simulink model "ASM_Traffic_V2X_Complete_Model_2"  (R2019a)
settings: Solver=ode1  StartTime=SIM.tstart.v  StopTime=Inf  FixedStep=SIM.StepSize.v  RelTol=1e-3
PostLoadFcn:
  | if any(exist('dsrtsu_mdlpostloadfcn', 'file') ~= 0), dsrtsu_mdlpostloadfcn('Execute', bdroot); end
  | try, asm_mdl_postloadfcn(bdroot, 'UpdateModel', 2200); catch, disp(lasterr); end,
undefined symbols (not defined in the file): _SensorPnts_1, _SensorPnts_13, _SensorPnts_17, _SensorPnts_21, _SensorPnts_25, _SensorPnts_29, _SensorPnts_33, _SensorPnts_37, _SensorPnts_41, _SensorPnts_45, _SensorPnts_49, _SensorPnts_5, _SensorPnts_53, _SensorPnts_57, _SensorPnts_9, _to_, CPT, G5A, ITS, MDL, rad, s_to_rpm, SIM
libraries: simulink x169, ASM_VehicleDynamics_lib x126, ASM_Traffic_lib x83, ASM_Utils_lib x49, mdbs x45, ASM_Environment_lib x17, dspindex x12, dsaV2xLibraryAux x10, dsmpblib x6, dsaV2xAsn1Library x4, dsaV2xLibrary x4, ASM_BrakeHydraulics_lib x4
(part 11 of 36)

== system ASM_Traffic_V2X_Complete_Model_2/MDL/Drivetrain/Transmission/AutomaticTransmission ==
  Ctrl_Lockup_Clutch[%] : Inport
  Gear[] : Inport  Port=2
  n_Engine[rad|s] : Inport  Port=3
  Trq_Engine[Nm] : Inport  Port=4
  omega_In_Diff[rad|s] : Inport  Port=5
  FROM_STABILIZATION_CLUTCH : Inport  Port=6
  Reset[0|1] : Inport  Port=7
  Enable : EnablePort  PropagateVarSize=During execution
  ASMSignalCollector : Subsystem
  GEARBOX_AT : ASM_VehicleDynamics_lib/Drivetrain/Gearbox/GEARBOX_AT  Tag=ASM_SUBCOMPONENT  Map_GearRatio=MDL.Drivetrain.AutomaticTransmission.Gearbox.Map_GearRatio  Const_SyncTime=MDL.Drivetrain.AutomaticTransmission.Gearbox.Const_SyncTime  Const_Inertia_InputGear=MDL.Drivetrain.AutomaticTransmission.Gearbox.Const_Inertia_InputGear  Const_Damping_InputGear=MDL.Drivetrain.AutomaticTransmission.Gearbox.Const_Damping_InputGear  Map_Inertia_Out=MDL.Drivetrain.AutomaticTransmission.Gearbox.Map_Inertia_Out  Map_Forward_Efficiency=MDL.Drivetrain.AutomaticTransmission.Gearbox.Map_Forward_Efficiency  Map_Reverse_Efficiency=MDL.Drivetrain.AutomaticTransmission.Gearbox.Map_Reverse_Efficiency  StepSize=SIM.StepSize  ASMProperties=struct('Name','GEARBOX_AT','Version','9.0','Library','ASM_VehicleDynamics_lib')  ASMInstanceName=gearbox_at  ASMInstanceID=1
  LOCKUP_CLUTCH : ASM_VehicleDynamics_lib/Drivetrain/Clutch/LOCKUP_CLUTCH  Tag=ASM_SUBCOMPONENT  Const_Torque_Max=MDL.Drivetrain.AutomaticTransmission.Clutch.Const_Torque_Max  Map_Trq_Clutch_Red=MDL.Drivetrain.AutomaticTransmission.Clutch.Map_Trq_Clutch_Red  Const_Coef_DynamicClutchTrq=MDL.Drivetrain.AutomaticTransmission.Clutch.Const_Coef_DynamicClutchTrq  Const_Inertia=MDL.Drivetrain.AutomaticTransmission.Clutch.Const_Inertia  StepSize=SIM.StepSize  ASMProperties=struct('Name','LOCKUP_CLUTCH','Version','5.0','Library','ASM_VehicleDynamics_lib')  ASMInstanceName=TorqueConverter  ASMInstanceID=1
  SignalConversion : SignalConversion  OverrideOpt=off
  TORQUE_CONVERTER : ASM_VehicleDynamics_lib/Drivetrain/Clutch/TORQUE_CONVERTER  Tag=ASM_SUBCOMPONENT  Map_Eta_Slip=MDL.Drivetrain.AutomaticTransmission.TorqueConverter.Map_Eta_Slip  Map_Rel_Trq_PumpTurb=MDL.Drivetrain.AutomaticTransmission.TorqueConverter.Map_Rel_Trq_PumpTurb  ASMProperties=struct('Name','TORQUE_CONVERTER','Version','6.0','Library','ASM_VehicleDynamics_lib')  ASMInstanceName=TorqueConverter  ASMInstanceID=1
  Torque_Summation : Subsystem
  omega_Out_ClutchPlate_Init[rad|s] : Constant  Value=0
  ASMSignalBus : Outport
  Trq_In_Converter[Nm] : Outport  Port=2
  Trq_Out_Trm[Nm] : Outport  Port=3
  Inertia_Out_Trm[kgm2] : Outport  Port=4
  TO_STABILIZATION_GEARBOX : Outport  Port=5
  TO_STABILIZATION_CLUTCH : Outport  Port=6
  TO_STABILIZATION_TORQUE_CONVERTER : Outport  Port=7
  tag scope: ASMBUS_Drivetrain_AutomaticTransmission_Gearbox=global, ASMBUS_Drivetrain_AutomaticTransmission_LockUpClutch=global, ASMBUS_Drivetrain_AutomaticTransmission_TorqueConverter=global
  wires:
  Reset[0|1]/1 -> LOCKUP_CLUTCH/6, GEARBOX_AT/4
  ASMSignalCollector/1(ASMSignalBus) -> ASMSignalBus/1
  TORQUE_CONVERTER/2 -> Torque_Summation/3(Trq_Pump[Nm])
  LOCKUP_CLUTCH/2 -> Torque_Summation/1(Trq_Fric[Nm])
  omega_In_Diff[rad|s]/1 -> GEARBOX_AT/3
  Gear[]/1 -> GEARBOX_AT/2
  GEARBOX_AT/4 -> Inertia_Out_Trm[kgm2]/1
  GEARBOX_AT/3 -> Trq_Out_Trm[Nm]/1
  GEARBOX_AT/2 -> LOCKUP_CLUTCH/5, TORQUE_CONVERTER/2
  FROM_STABILIZATION_CLUTCH/1 -> LOCKUP_CLUTCH/4
  Ctrl_Lockup_Clutch[%]/1 -> LOCKUP_CLUTCH/3
  Trq_Engine[Nm]/1 -> LOCKUP_CLUTCH/2
  n_Engine[rad|s]/1 -> LOCKUP_CLUTCH/1, TORQUE_CONVERTER/1
  TORQUE_CONVERTER/1 -> [ASMBUS_Drivetrain_AutomaticTransmission_TorqueConverter]
  LOCKUP_CLUTCH/3 -> Torque_Summation/2(Trq_Out_LockupClutch[Nm])
  TORQUE_CONVERTER/3 -> Torque_Summation/4(Trq_Turbine[Nm])
  Torque_Summation/1(Trq_In_Converter[Nm]) -> Trq_In_Converter[Nm]/1
  Torque_Summation/2(Trq_In_Trm[Nm]) -> GEARBOX_AT/1
  GEARBOX_AT/1 -> [ASMBUS_Drivetrain_AutomaticTransmission_Gearbox]
  LOCKUP_CLUTCH/1 -> [ASMBUS_Drivetrain_AutomaticTransmission_LockUpClutch]
  GEARBOX_AT/5 -> SignalConversion/1
  TORQUE_CONVERTER/4 -> TO_STABILIZATION_TORQUE_CONVERTER/1
  LOCKUP_CLUTCH/4 -> TO_STABILIZATION_CLUTCH/1
  omega_Out_ClutchPlate_Init[rad|s]/1 -> LOCKUP_CLUTCH/7
  SignalConversion/1 -> TO_STABILIZATION_GEARBOX/1

== system ASM_Traffic_V2X_Complete_Model_2/MDL/Drivetrain/Transmission/ManualTransmission ==
  Pos_Clutch[%] : Inport
  Gear[] : Inport  Port=2
  n_Engine[rad|s] : Inport  Port=3
  Trq_Engine[Nm] : Inport  Port=4
  omega_In_Diff[rad|s] : Inport  Port=5
  FROM_STABILIZATION_CLUTCH : Inport  Port=6
  Reset[0|1] : Inport  Port=7
  Enable : EnablePort  PropagateVarSize=During execution
  ASMSignalCollector : Subsystem
  CLUTCH : ASM_VehicleDynamics_lib/Drivetrain/Clutch/CLUTCH  Tag=ASM_SUBCOMPONENT  Map_Stiffness=MDL.Drivetrain.ManualTransmission.Clutch.Map_Stiffness  Const_Damping=MDL.Drivetrain.ManualTransmission.Clutch.Const_Damping  Const_Torque_Max=MDL.Drivetrain.ManualTransmission.Clutch.Const_Torque_Max  Map_Trq_Clutch_Red=MDL.Drivetrain.ManualTransmission.Clutch.Map_Trq_Clutch_Red  Const_Coef_DynamicClutchTrq=MDL.Drivetrain.ManualTransmission.Clutch.Const_Coef_DynamicClutchTrq  Const_Inertia=MDL.Drivetrain.ManualTransmission.Clutch.Const_Inertia  StepSize=SIM.StepSize  ASMProperties=struct('Name','CLUTCH','Version','7.0','Library','ASM_VehicleDynamics_lib')  ASMInstanceName=clutch  ASMInstanceID=1
  GEARBOX_MT : ASM_VehicleDynamics_lib/Drivetrain/Gearbox/GEARBOX_MT  Tag=ASM_SUBCOMPONENT  Map_GearRatio=MDL.Drivetrain.ManualTransmission.Gearbox.Map_GearRatio  Const_SyncTime=MDL.Drivetrain.ManualTransmission.Gearbox.Const_SyncTime  Const_Inertia_InputGear=MDL.Drivetrain.ManualTransmission.Gearbox.Const_Inertia_InputGear  Const_Damping_InputGear=MDL.Drivetrain.ManualTransmission.Gearbox.Const_Damping_InputGear  Map_Inertia_Out=MDL.Drivetrain.ManualTransmission.Gearbox.Map_Inertia_Out  Map_Forward_Efficiency=MDL.Drivetrain.ManualTransmission.Gearbox.Map_Forward_Efficiency  Map_Reverse_Efficiency=MDL.Drivetrain.ManualTransmission.Gearbox.Map_Reverse_Efficiency  StepSize=SIM.StepSize  ASMProperties=struct('Name','GEARBOX_MT','Version','9.0','Library','ASM_VehicleDynamics_lib')  ASMInstanceName=gearbox_mt  ASMInstanceID=1
  SignalConversion : SignalConversion  OverrideOpt=off
  omega_Out_ClutchPlate_Init[rad|s] : Constant  Value=0
  ASMSignalBus : Outport
  Trq_Fric[Nm] : Outport  Port=2
  Trq_Out_Trm[Nm] : Outport  Port=3
  Inertia_Out_Trm[kgm2] : Outport  Port=4
  TO_STABILIZATION_GEARBOX : Outport  Port=5
  TO_STABILIZATION_CLUTCH : Outport  Port=6
  tag scope: ASMBUS_Drivetrain_ManualTransmission_Clutch=global, ASMBUS_Drivetrain_ManualTransmission_Gearbox=global
  wires:
  Reset[0|1]/1 -> GEARBOX_MT/4, CLUTCH/6
  ASMSignalCollector/1(ASMSignalBus) -> ASMSignalBus/1
  CLUTCH/3 -> GEARBOX_MT/1
  GEARBOX_MT/2 -> CLUTCH/5
  GEARBOX_MT/3 -> Trq_Out_Trm[Nm]/1
  GEARBOX_MT/4 -> Inertia_Out_Trm[kgm2]/1
  omega_In_Diff[rad|s]/1 -> GEARBOX_MT/3
  Gear[]/1 -> GEARBOX_MT/2
  n_Engine[rad|s]/1 -> CLUTCH/1
  Trq_Engine[Nm]/1 -> CLUTCH/2
  Pos_Clutch[%]/1 -> CLUTCH/3
  FROM_STABILIZATION_CLUTCH/1 -> CLUTCH/4
  GEARBOX_MT/1 -> [ASMBUS_Drivetrain_ManualTransmission_Gearbox]
  GEARBOX_MT/5 -> SignalConversion/1
  CLUTCH/4 -> TO_STABILIZATION_CLUTCH/1
  CLUTCH/1 -> [ASMBUS_Drivetrain_ManualTransmission_Clutch]
  CLUTCH/2 -> Trq_Fric[Nm]/1
  omega_Out_ClutchPlate_Init[rad|s]/1 -> CLUTCH/7
  SignalConversion/1 -> TO_STABILIZATION_GEARBOX/1

== system ASM_Traffic_V2X_Complete_Model_2/MDL/Environment/Driver/ASMSignalCollector ==
  Bus Creator : BusCreator  Inputs=4
  tag scope: ASMBUS_Environment_Driver=global
  wires:
  [ASMBUS_Env_Driver_SignalSelection] -> Bus Creator/1
  [ASMBUS_Env_Driver_LatController] -> Bus Creator/4
  [ASMBUS_Env_Driver_vRef] -> Bus Creator/3
  [ASMBUS_Env_Driver_LongController] -> Bus Creator/2
  Bus Creator/1 -> [ASMBUS_Environment_Driver]  "Driver"

== system ASM_Traffic_V2X_Complete_Model_2/MDL/Environment/Driver/LateralController ==
  Maneuver_Signals : Inport
  VehicleDynamics_Signals : Inport  Port=2
  Road_Signals : Inport  Port=3
  ASMSignalCollector : Subsystem
  Bus Creator : BusCreator  Inputs=2
  Bus Selector1 : BusSelector  OutputSignals=ModeSignals.LatDriver[1LatCtrl1|2LatCtrl2],ModeSignals.Steer_Mode[1Stim|2Driver|3Fix]
  Bus Selector2 : BusSelector  OutputSignals=Road_ASMVeh.Angle_Yaw_Veh_Road[deg],Road_ASMVeh.Pos_x_Ref_Veh_Road[m],Road_Preview.Pos_x_Preview_Road[m],Road_ASMVeh.Pos_y_Ref_Veh_Road[m],Road_Preview.Pos_y_Preview_Road[m],Road_ASMVeh.Curv_Veh_Road[1|m]
  Bus Selector3 : BusSelector  OutputSignals=VehicleMovement.Velocities.v_x_Vehicle[km|h],VehicleMovement.Velocities.v_y_Vehicle[km|h],VehicleMovement.Positions.Angle_Vehicle_CoorSys_E[x;y;z][deg].Angle_Yaw_Vehicle_CoorSys_E[deg],VehicleMovement.Velocities.YawRate_Vehicle[deg|s],VehicleMovement.Positions.Pos_Vehicle_CoorSys_E[x;y;z][m].Pos_x_Vehicle_CoorSys_E[m],VehicleMovement.Positions.Pos_Vehicle_CoorSys_E[x;y;z][m].Pos_y_Vehicle_CoorSys_E[m],Steering.i_Steering_Mean[],Tire.CorneringStiffness_Tire_Front[N|rad],Tire.CorneringStiffness_Tire_Rear[N|rad],VehicleMovement.Parameters.m_TotalVehicle[kg],VehicleMovement.Parameters.Pos_x_CoG_Vehicle_Total[m],VehicleMovement.Parameters.Inertia_z_Vehicle_Total[kgm2]
  Bus Selector4 : BusSelector  OutputSignals=Parameters.Width_Deadzone_LatCtrl[m],MdlControl.Reset_VehicleStates[0|1],ModeSignals.Steer_Mode[1Stim|2Driver|3Fix],RefSignals.Angle_SteeringWheel_Maneuver[deg],ModeSignals.LatCtrl_Mode[1Pos|2Yaw]
  LATERAL_CONTROL1 : ASM_Environment_lib/Environment/Driver/LATERAL_CONTROL1  Tag=ASM_SUBCOMPONENT  Const_t_Preview_LatCtrl=MDL.Environment.Driver.LateralController.LateralControl1.Const_t_Preview_LatCtrl  Const_t_PT1_LatCtrl=MDL.Environment.Driver.LateralController.LateralControl1.Const_t_PT1_LatCtrl  Const_WheelBase=MDL.Environment.Driver.LateralController.LateralControl1.Const_WheelBase  StepSize=SIM.StepSize  ASMProperties=struct('Name','LATERAL_CONTROL1','Version','13.0','Library','ASM_Environment_lib')  ASMInstanceName=lateral_control1  ASMInstanceID=1
  LATERAL_CONTROL2 : ASM_Environment_lib/Environment/Driver/LATERAL_CONTROL2  Tag=ASM_SUBCOMPONENT  Const_LatCtrl_kLat=MDL.Environment.Driver.LateralController.LateralControl2.Const_LatCtrl_kLat  Const_LatCtrl_kLat_i=MDL.Environment.Driver.LateralController.LateralControl2.Const_LatCtrl_kLat_i  Const_LatCtrl_kLat_Preview=MDL.Environment.Driver.LateralController.LateralControl2.Const_LatCtrl_kLat_Preview  Const_LatCtrl_kYaw=MDL.Environment.Driver.LateralController.LateralControl2.Const_LatCtrl_kYaw  Const_t_Preview_LatCtrl=MDL.Environment.Driver.LateralController.LateralControl2.Const_t_Preview_LatCtrl  Const_t_PT1_LatCtrl=MDL.Environment.Driver.LateralController.LateralControl2.Const_t_PT1_LatCtrl  Const_Kp_YawRate_Ctrl=MDL.Environment.Driver.LateralController.LateralControl2.Const_Kp_YawRate_Ctrl  Const_Ki_YawRate_Ctrl=MDL.Environment.Driver.LateralController.LateralControl2.Const_Ki_YawRate_Ctrl  StepSize=SIM.StepSize  ASMProperties=struct('Name','LATERAL_CONTROL2','Version','8.0','Library','ASM_Environment_lib')  ASMInstanceName=lateral_control2  ASMInstanceID=1
  LatCtrl1_Enable : Fcn  Expr=(u(1) == 1) * (u(2) == 2)
  LatCtrl2_Enable : Fcn  Expr=(u(1) == 2) * (u(2) == 2)
  Memory : Memory
  Multiport Switch : MultiPortSwitch  Inputs=2  SaturateOnIntegerOverflow=on
  Multiport Switch1 : MultiPortSwitch  Inputs=2  SaturateOnIntegerOverflow=on
  Mux2 : Mux  Inputs=2
  POSITION_ERRORS : ASM_Environment_lib/Environment/Driver/POSITION_ERRORS  Tag=ASM_SUBCOMPONENT  ASMProperties=struct('Name','POSITION_ERRORS','Version','1.0','Library','ASM_Environment_lib')  ASMInstanceName=position_errors  ASMInstanceID=1
  UnitConversion1 : ASM_Utils_lib/UnitConversion/UnitConversion  Selection=km/h_to_m/s
  UnitConversion2 : ASM_Utils_lib/UnitConversion/UnitConversion  Selection=km/h_to_m/s
  UnitConversion3 : ASM_Utils_lib/UnitConversion/UnitConversion  Selection=deg_to_rad
  Y_pos : Display
  laneNum : Display
  laneNumber : MATLAB Function  TreatAsAtomicUnit=on
  s_Preview_LatCtrl[m] : Outport
  Angle_SteeringWheel_LatCtrl[deg] : Outport  Port=2
  tag scope: ASMBUS_Env_Driver_LatCtrl1=global, ASMBUS_Env_Driver_LatCtrl2=global, ASMBUS_Env_Driver_LatCtrl_PosError=global
  wires:
  LatCtrl2_Enable/1 -> LATERAL_CONTROL2/1
  Bus Selector4/5 -> LATERAL_CONTROL2/18  "<LatCtrl_Mode[1Pos|2Yaw]>"
  Bus Selector2/6 -> LATERAL_CONTROL2/19  "<Curv_Veh_Road[1|m]>"
  Road_Signals/1 -> Bus Selector2/1
  Bus Selector2/1 -> LATERAL_CONTROL2/7  "<Angle_Yaw_Veh_Road[deg]>"
  Bus Selector4/4 -> LATERAL_CONTROL1/20, LATERAL_CONTROL2/16  "<Angle_SteeringWheel_Maneuver[deg]>"
  Bus Selector4/3 -> LATERAL_CONTROL1/19, LATERAL_CONTROL2/15  "<Steer_Mode[1Stim|2Driver|3Fix]>"
  Bus Selector4/2 -> LATERAL_CONTROL1/18, LATERAL_CONTROL2/14  "<Reset_VehicleStates[0|1]>"
  Bus Selector4/1 -> LATERAL_CONTROL1/17, LATERAL_CONTROL2/13  "<Width_Deadzone_LatCtrl[m]>"
  Bus Selector3/12 -> LATERAL_CONTROL1/16  "<Inertia_z_Vehicle_Total[kgm2]>"
  Bus Selector3/11 -> LATERAL_CONTROL1/15  "<Pos_x_CoG_Vehicle_Total[m]>"
  Bus Selector3/10 -> LATERAL_CONTROL1/14  "<m_TotalVehicle[kg]>"
  Memory/1 -> LATERAL_CONTROL1/13, LATERAL_CONTROL2/12
  Multiport Switch1/1 -> Memory/1, ASMSignalCollector/2(Angle_SteeringWheel_LatCtrl[deg]), Angle_SteeringWheel_LatCtrl[deg]/1
  UnitConversion3/1 -> LATERAL_CONTROL1/5, LATERAL_CONTROL2/17
  UnitConversion1/1 -> LATERAL_CONTROL1/2, LATERAL_CONTROL2/3
  LatCtrl1_Enable/1 -> LATERAL_CONTROL1/1
  Bus Selector3/4 -> UnitConversion3/1  "<YawRate_Vehicle[deg|s]>"
  Mux2/1 -> LatCtrl2_Enable/1, LatCtrl1_Enable/1
  Bus Selector1/2 -> Mux2/2  "<Steer_Mode[1Stim|2Driver|3Fix]>"
  Bus Selector3/9 -> LATERAL_CONTROL1/10  "<CorneringStiffness_Tire_Rear[N|rad]>"
  Bus Selector3/8 -> LATERAL_CONTROL1/9  "<CorneringStiffness_Tire_Front[N|rad]>"
  Bus Selector3/7 -> LATERAL_CONTROL1/8, LATERAL_CONTROL2/2  "<i_Steering_Mean[]>"
  POSITION_ERRORS/1 -> [ASMBUS_Env_Driver_LatCtrl_PosError]
  POSITION_ERRORS/2 -> ASMSignalCollector/3(e_Lat[m])
  LATERAL_CONTROL2/1 -> [ASMBUS_Env_Driver_LatCtrl2]
  LATERAL_CONTROL2/3 -> Multiport Switch1/3
  Bus Selector1/1 -> Mux2/1, Multiport Switch/1, Multiport Switch1/1  "<LatDriver[1LatCtrl1|2LatCtrl2]>"
  Maneuver_Signals/1 -> Bus Selector1/1, Bus Selector4/1
  UnitConversion2/1 -> LATERAL_CONTROL1/3
  Bus Selector3/5 -> LATERAL_CONTROL1/6, POSITION_ERRORS/2, LATERAL_CONTROL2/5  "<Pos_x_Vehicle_CoorSys_E[m]>"
  Bus Selector3/3 -> LATERAL_CONTROL1/4, POSITION_ERRORS/1, LATERAL_CONTROL2/4  "<Angle_Yaw_Vehicle_CoorSys_E[deg]>"
  Bus Selector3/2 -> UnitConversion2/1  "<v_y_Vehicle[km|h]>"
  Bus Selector3/1 -> UnitConversion1/1  "<v_x_Vehicle[km|h]>"
  Bus Selector2/4 -> LATERAL_CONTROL2/10, POSITION_ERRORS/5  "<Pos_y_Ref_Veh_Road[m]>"
  Bus Selector2/2 -> LATERAL_CONTROL2/8, POSITION_ERRORS/4  "<Pos_x_Ref_Veh_Road[m]>"
  VehicleDynamics_Signals/1 -> Bus Selector3/1
  LATERAL_CONTROL1/3 -> Multiport Switch1/2
  LATERAL_CONTROL1/2 -> Multiport Switch/2
  LATERAL_CONTROL2/2 -> Multiport Switch/3
  Multiport Switch/1 -> ASMSignalCollector/1(s_Preview_LatCtrl[m]), s_Preview_LatCtrl[m]/1
  Bus Selector2/5 -> LATERAL_CONTROL1/12, LATERAL_CONTROL2/11  "<Pos_y_Preview_Road[m]>"
  Bus Selector2/3 -> LATERAL_CONTROL1/11, LATERAL_CONTROL2/9  "<Pos_x_Preview_Road[m]>"
  laneNumber/1(laneNumber) -> Bus Creator/1, laneNum/1
  LATERAL_CONTROL1/1 -> Bus Creator/2
  Bus Selector3/6 -> Y_pos/1, laneNumber/1(u), LATERAL_CONTROL1/7, POSITION_ERRORS/3, LATERAL_CONTROL2/6  "<Pos_y_Vehicle_CoorSys_E[m]>"
  Bus Creator/1 -> [ASMBUS_Env_Driver_LatCtrl1]

== system ASM_Traffic_V2X_Complete_Model_2/MDL/Environment/Driver/LongitudinalController ==
  Maneuver_Signals : Inport
  Drivetrain_Signals : Inport  Port=2
  SoftECU_Engine_Signals : Inport  Port=3
  VehicleDynamics_Signals : Inport  Port=4
  v_Vehicle_Ref[m|s] : Inport  Port=5
  v_Vehicle_Ref_Preview[m|s] : Inport  Port=6
  ASMSignalCollector : Subsystem
  Bus Selector1 : BusSelector  OutputSignals=Parameters.Gear_Max[],RefSignals.Pos_AccPedal_Maneuver[%],RefSignals.Pos_BrakePedal_Maneuver[%],ModeSignals.AccBr_Mode[1Stim|2Driver],RefSignals.Gear_Maneuver[],RefSignals.Pos_ClutchPedal_Maneuver[%],ModeSignals.GearClutch_Mode[1Stim|2Driver|3OpenClutch|4RefGear],RefSignals.SelectorLever_Maneuver[],ModeSignals.SelectorLever_Mode[1Stim|2Driver],MdlControl.Reset_VehicleStates[0|1]
  Bus Selector2 : BusSelector  OutputSignals=VehicleMovement.Parameters.m_TotalVehicle[kg]
  Bus Selector3 : BusSelector  OutputSignals=n_Engine[rpm],omega_Out_Trm[rad|s]
  Bus Selector4 : BusSelector  OutputSignals=VehicleMovement.Velocities.v_x_Vehicle[km|h]
  Bus Selector5 : BusSelector  OutputSignals=SoftECU_Engine.State_Engine[0|1|2|3|4],SoftECU_Engine.Const_n_Engine_Idle_Set[rpm]
  Bus Selector6 : BusSelector  OutputSignals=ModeSignals.AccBr_Mode[1Stim|2Driver],RefSignals.Pos_AccPedal_Maneuver[%],RefSignals.Pos_BrakePedal_Maneuver[%],MdlControl.Reset_VehicleStates[0|1]
  Default_GearClutch_Mode : Subsystem
      mask Display: disp('Default GearClutch_Mode')
  Driving_Resistances : Subsystem
  GEAR_SHIFTER : ASM_Environment_lib/Environment/Driver/GEAR_SHIFTER  Tag=ASM_SUBCOMPONENT  Map_Gear_StartUp=MDL.Environment.Driver.LongitudinalController.GearShifter.Map_Gear_StartUp  Const_n_Engine_StartUp_Set=MDL.Environment.Driver.LongitudinalController.GearShifter.Const_n_Engine_StartUp_Set  Const_P_Gain_StartUp=MDL.Environment.Driver.LongitudinalController.GearShifter.Const_P_Gain_StartUp  Const_I_Gain_StartUp=MDL.Environment.Driver.LongitudinalController.GearShifter.Const_I_Gain_StartUp  Const_D_Gain_StartUp=MDL.Environment.Driver.LongitudinalController.GearShifter.Const_D_Gain_StartUp  Const_a_x_Vehicle_UpLim=MDL.Environment.Driver.LongitudinalController.GearShifter.Const_a_x_Vehicle_UpLim  Const_a_Tractive_Res_UpLim=MDL.Environment.Driver.LongitudinalController.GearShifter.Const_a_Tractive_Res_UpLim  Const_v_x_Vehicle_LowLim=MDL.Environment.Driver.LongitudinalController.GearShifter.Const_v_x_Vehicle_LowLim  Const_a_x_Vehicle_LowLim=MDL.Environment.Driver.LongitudinalController.GearShifter.Const_a_x_Vehicle_LowLim  Const_t_Gear_Neutral=MDL.Environment.Driver.LongitudinalController.GearShifter.Const_t_Gear_Neutral  Const_t_Hold_ClutchPedal=MDL.Environment.Driver.LongitudinalController.GearShifter.Const_t_Hold_ClutchPedal  Map_Pos_AccPedal=MDL.Environment.Driver.LongitudinalController.GearShifter.Map_Pos_AccPedal  Const_P_Gain_ClutchPedal=MDL.Environment.Driver.LongitudinalController.GearShifter.Const_P_Gain_ClutchPedal  Const_I_Gain_ClutchPedal=MDL.Environment.Driver.LongitudinalController.GearShifter.Const_I_Gain_ClutchPedal  Map_Pos_ClutchPedal_Disengagement_StartUp=MDL.Environment.Driver.LongitudinalController.GearShifter.Map_Pos_ClutchPedal_Disengagement_StartUp  Map_Pos_ClutchPedal_Disengagement=MDL.Environment.Driver.LongitudinalController.GearShifter.Map_Pos_ClutchPedal_Disengagement  Map_Pos_ClutchPedal_Engagement_StartUp=MDL.Environment.Driver.LongitudinalController.GearShifter.Map_Pos_ClutchPedal_Engagement_StartUp  Map_Pos_ClutchPedal_Engagement=MDL.Environment.Driver.LongitudinalController.GearShifter.Map_Pos_ClutchPedal_Engagement  Map_n_Engine_Upshift_Lim=MDL.Environment.Driver.LongitudinalController.GearShifter.Map_n_Engine_Upshift_Lim  Map_n_Engine_Downshift_Lim=MDL.Environment.Driver.LongitudinalController.GearShifter.Map_n_Engine_Downshift_Lim  Map_omega_Out_Trm_Shift_Bias=MDL.Environment.Driver.LongitudinalController.GearShifter.Map_omega_Out_Trm_Shift_Bias  Map_i_Ratio=MDL.Environment.Driver.LongitudinalController.GearShifter.Map_i_Ratio  Sw_Upshift_Gear_Skipping=MDL.Environment.Driver.LongitudinalController.GearShifter.Sw_Upshift_Gear_Skipping  Sw_ClutchPedal_EngineOff=MDL.Environment.Driver.LongitudinalController.GearShifter.Sw_ClutchPedal_EngineOff  StepSize=SIM.StepSize  ASMProperties=struct('Name','GEAR_SHIFTER','Version','17.0','Library','ASM_Environment_lib')  ASMInstanceName=gear_shifter  ASMInstanceID=1
  Gear_Min_Maneuver[0Off|-n_-1] : Constant  Value=0
  LONGITUDINAL_CONTROL : ASM_Environment_lib/Environment/Driver/LONGITUDINAL_CONTROL  Tag=ASM_SUBCOMPONENT  Map_P_vCtrl=MDL.Environment.Driver.LongitudinalController.LongControl.Map_P_vCtrl  Map_I_vCtrl=MDL.Environment.Driver.LongitudinalController.LongControl.Map_I_vCtrl  Const_P_FeedForward_aCtrl=MDL.Environment.Driver.LongitudinalController.LongControl.Const_P_FeedForward_aCtrl  Const_Pos_BrakePedal_Standstill=MDL.Environment.Driver.LongitudinalController.LongControl.Const_Pos_BrakePedal_Standstill  Const_t_Min_Pedals=MDL.Environment.Driver.LongitudinalController.LongControl.Const_t_Min_Pedals  Const_Max_AccPedal=MDL.Environment.Driver.LongitudinalController.LongControl.Const_Max_AccPedal  Const_Rate_Rise_Max_AccPedal=MDL.Environment.Driver.LongitudinalController.LongControl.Const_Rate_Rise_Max_AccPedal  Const_Rate_Drop_Max_AccPedal=MDL.Environment.Driver.LongitudinalController.LongControl.Const_Rate_Drop_Max_AccPedal  Const_Max_BrakePedal=MDL.Environment.Driver.LongitudinalController.LongControl.Const_Max_BrakePedal  Const_Rate_Rise_Max_BrakePedal=MDL.Environment.Driver.LongitudinalController.LongControl.Const_Rate_Rise_Max_BrakePedal  Const_Rate_Drop_Max_BrakePedal=MDL.Environment.Driver.LongitudinalController.LongControl.Const_Rate_Drop_Max_BrakePedal  Const_t_Preview=MDL.Environment.Driver.LongitudinalController.LongControl.Const_t_Preview  StepSize=SIM.StepSize  ASMProperties=struct('Name','LONGITUDINAL_CONTROL','Version','3.0','Library','ASM_Environment_lib')  ASMInstanceName=longitudinal_control  ASMInstanceID=1
  No_StartStop : Constant
  Running_Engine : Constant  Value=3
  UnitConversion : ASM_Utils_lib/UnitConversion/UnitConversion  Selection=km/h_to_m/s
  Pos_AccPedal[%] : Outport
  Pos_BrakePedal[%] : Outport  Port=2
  Pos_ClutchPedal[%] : Outport  Port=3
  Gear[] : Outport  Port=4
  SelectorLever[-3T|-2P|-1R|0N|1D] : Outport  Port=5
  t_Preview_vRef[s] : Outport  Port=6
  tag scope: ASMBUS_Env_Driver_GearShifter=global, ASMBUS_Env_Driver_LongCtrl=global
  wires:
  Running_Engine/1 -> LONGITUDINAL_CONTROL/8
  LONGITUDINAL_CONTROL/2 -> t_Preview_vRef[s]/1
  v_Vehicle_Ref_Preview[m|s]/1 -> GEAR_SHIFTER/24, LONGITUDINAL_CONTROL/3
  Bus Selector6/4 -> LONGITUDINAL_CONTROL/7  "<Reset_VehicleStates[0|1]>"
  Bus Selector6/3 -> LONGITUDINAL_CONTROL/6  "<Pos_BrakePedal_Maneuver[%]>"
  Bus Selector6/2 -> LONGITUDINAL_CONTROL/5  "<Pos_AccPedal_Maneuver[%]>"
  Bus Selector6/1 -> LONGITUDINAL_CONTROL/4  "<AccBr_Mode[1Stim|2Driver]>"
  Bus Selector3/2 -> GEAR_SHIFTER/9  "<omega_Out_Trm[rad|s]>"
  Driving_Resistances/1(F_Tractive_Res[N]) -> GEAR_SHIFTER/4
  No_StartStop/1 -> GEAR_SHIFTER/23, LONGITUDINAL_CONTROL/9
  Default_GearClutch_Mode/1(GearClutch_Mode[1Stim|2Driver|3OpenClutch|4RefGear]_) -> GEAR_SHIFTER/19
  GEAR_SHIFTER/6 -> SelectorLever[-3T|-2P|-1R|0N|1D]/1
  GEAR_SHIFTER/5 -> Gear[]/1
  GEAR_SHIFTER/4 -> Pos_ClutchPedal[%]/1
  GEAR_SHIFTER/3 -> Pos_BrakePedal[%]/1
  GEAR_SHIFTER/2 -> Pos_AccPedal[%]/1
  Bus Selector1/9 -> GEAR_SHIFTER/21  "<SelectorLever_Mode[1Stim|2Driver]>"
  Bus Selector1/8 -> GEAR_SHIFTER/20  "<SelectorLever_Maneuver[]>"
  Bus Selector1/7 -> Default_GearClutch_Mode/1(GearClutch_Mode[1Stim|2Driver|3OpenClutch|4RefGear])  "<GearClutch_Mode[1Stim|2Driver|3OpenClutch|4RefGear]>"
  Bus Selector1/6 -> GEAR_SHIFTER/18  "<Pos_ClutchPedal_Maneuver[%]>"
  Bus Selector1/5 -> GEAR_SHIFTER/17  "<Gear_Maneuver[]>"
  Bus Selector1/4 -> GEAR_SHIFTER/16  "<AccBr_Mode[1Stim|2Driver]>"
  Bus Selector1/3 -> GEAR_SHIFTER/15  "<Pos_BrakePedal_Maneuver[%]>"
  Bus Selector1/2 -> GEAR_SHIFTER/14  "<Pos_AccPedal_Maneuver[%]>"
  Bus Selector1/1 -> GEAR_SHIFTER/13  "<Gear_Max[]>"
  Bus Selector5/2 -> GEAR_SHIFTER/11  "<Const_n_Engine_Idle_Set[rpm]>"
  Bus Selector5/1 -> GEAR_SHIFTER/10  "<State_Engine[0|1|2|3|4]>"
  Gear_Min_Maneuver[0Off|-n_-1]/1 -> GEAR_SHIFTER/12
  LONGITUDINAL_CONTROL/3 -> GEAR_SHIFTER/2
  GEAR_SHIFTER/1 -> [ASMBUS_Env_Driver_GearShifter]
  LONGITUDINAL_CONTROL/1 -> [ASMBUS_Env_Driver_LongCtrl]
  SoftECU_Engine_Signals/1 -> Bus Selector5/1
  Bus Selector1/10 -> GEAR_SHIFTER/22  "<Reset_VehicleStates[0|1]>"
  Bus Selector2/1 -> GEAR_SHIFTER/8  "<m_TotalVehicle[kg]>"
  UnitConversion/1 -> GEAR_SHIFTER/5, LONGITUDINAL_CONTROL/1
  Maneuver_Signals/1 -> Bus Selector6/1, Bus Selector1/1
  Bus Selector3/1 -> GEAR_SHIFTER/7  "<n_Engine[rpm]>"
  Drivetrain_Signals/1 -> Bus Selector3/1
  LONGITUDINAL_CONTROL/4 -> GEAR_SHIFTER/3
  [TAG_Sw_Transmission_Mode] -> GEAR_SHIFTER/1
  Bus Selector4/1 -> UnitConversion/1  "<v_x_Vehicle[km|h]>"
  VehicleDynamics_Signals/1 -> Bus Selector4/1, Bus Selector2/1, Driving_Resistances/1(VehicleDynamics_Signals)
  v_Vehicle_Ref[m|s]/1 -> GEAR_SHIFTER/6, LONGITUDINAL_CONTROL/2

== system ASM_Traffic_V2X_Complete_Model_2/MDL/Environment/Driver/ReferenceVelocity ==
  Maneuver_Signals : Inport
  VehicleDynamics_Signals : Inport  Port=2
  Road_Signals : Inport  Port=3
  Bus Selector1 : BusSelector  OutputSignals=RefSignals.v_Vehicle_Ref_Preview_Maneuver[m|s]
  Bus Selector2 : BusSelector  OutputSignals=VehicleMovement.Velocities.v_x_Vehicle[km|h]
  Bus Selector3 : BusSelector  OutputSignals=MdlControl.Reset_VehicleStates[0|1],ModeSignals.AccBr_Mode[1Stim|2Driver]
  Bus Selector4 : BusSelector  OutputSignals=Road_ASMVeh.s_Veh_Road[m],Road_Preview.Pitch_Preview_Road[deg],Road_Preview.Pos_z_Preview_Road[m]
  Bus Selector5 : BusSelector  OutputSignals=Road_Info.Speed_Limit_Veh[km|h],Road_Preview.Speed_Limit_Preview_Road[km|h]
  Bus Selector6 : BusSelector  OutputSignals=Road_Info.Dist_Border_Left[m],Road_Info.Dist_Border_Right[m]
  Bus Selector7 : BusSelector  OutputSignals=Road_Preview.x_Preview_DriverCurv[m],Road_Preview.y_Preview_DriverCurv[m],Road_ASMVeh.Curv_Veh_Road[1|m],Road_Preview.Curv_Preview_Road[1|m]
  Bus Selector8 : BusSelector  OutputSignals=ModeSignals.AdaptVelocityToRoad_Mode[1Off|2On],RefSignals.v_Vehicle_Ref_Maneuver[m|s],Parameters.a_x_Max[m|s2],Parameters.a_x_Brake_Threshold[m|s2],Parameters.a_y_Max[m|s2]
  Bus Selector9 : BusSelector  OutputSignals=ModeSignals.CurvatureCalculation_Mode[1Road|2Driver]
  Curves_are_not_considered : Gain
  DRIVER_CURVATURE : ASM_Environment_lib/Environment/Driver/DRIVER_CURVATURE  Tag=ASM_SUBCOMPONENT  ASMProperties=struct('Name','DRIVER_CURVATURE','Version','1.0','Library','ASM_Environment_lib')  ASMInstanceName=driver_curvature  ASMInstanceID=1
  Extend_Dimension : Subsystem
  Reduce_Dimension2 : Subsystem
  Reduce_Dimension3 : Subsystem
  Reduce_Dimension4 : Subsystem
  Reduce_Dimension5 : Subsystem
  Terminator : Terminator
  Terminator_2 : Terminator
  UnitConversion : ASM_Utils_lib/UnitConversion/UnitConversion  Selection=km/h_to_m/s
  UnitConversion1 : ASM_Utils_lib/UnitConversion/UnitConversion  Selection=km/h_to_m/s
  UnitConversion4 : ASM_Utils_lib/UnitConversion/UnitConversion  Selection=km/h_to_m/s
  V_ROAD_REF : ASM_Environment_lib/Environment/Driver/V_ROAD_REF  Tag=ASM_SUBCOMPONENT  StepSize=SIM.StepSize  ASMProperties=struct('Name','V_ROAD_REF','Version','7.0','Library','ASM_Environment_lib')  ASMInstanceName=v_road_ref  ASMInstanceID=1
  a_z_Max_Deflect[m|s2] : Constant  Value=2.5
  a_z_Max_Rebound[m|s2] : Constant  Value=-3.5
  v_Vehicle_Ref[m|s] : Outport
  v_Vehicle_Ref_Preview[m|s] : Outport  Port=2
  s_Preview_vRef[m] : Outport  Port=3
  tag scope: ASMBUS_Env_Driver_GetCurvature=global, ASMBUS_Env_Driver_vRef=global
  wires:
  Reduce_Dimension5/1(Out) -> DRIVER_CURVATURE/5
  Bus Selector7/1 -> DRIVER_CURVATURE/2  "<x_Preview_DriverCurv[m]>"
  Bus Selector7/2 -> DRIVER_CURVATURE/3  "<y_Preview_DriverCurv[m]>"
  Bus Selector7/4 -> Reduce_Dimension5/1(In)  "<Curv_Preview_Road[1|m]>"
  Bus Selector7/3 -> DRIVER_CURVATURE/4  "<Curv_Veh_Road[1|m]>"
  Road_Signals/1 -> Bus Selector5/1, Bus Selector4/1, Bus Selector6/1, Bus Selector7/1
  Maneuver_Signals/1 -> Bus Selector1/1, Bus Selector9/1, Bus Selector3/1, Bus Selector8/1
  Bus Selector9/1 -> DRIVER_CURVATURE/1  "<CurvatureCalculation_Mode[1Road|2Driver]>"
  [ASMBUS_Env_Driver_GetCurvature] -> Terminator_2/1
  DRIVER_CURVATURE/3 -> V_ROAD_REF/8
  DRIVER_CURVATURE/2 -> V_ROAD_REF/7
  DRIVER_CURVATURE/1 -> [ASMBUS_Env_Driver_GetCurvature]
  Bus Selector6/2 -> V_ROAD_REF/19  "<Dist_Border_Right[m]>"
  Bus Selector6/1 -> V_ROAD_REF/18  "<Dist_Border_Left[m]>"
  V_ROAD_REF/4 -> Extend_Dimension/1(In)
  V_ROAD_REF/3 -> v_Vehicle_Ref[m|s]/1
  V_ROAD_REF/2 -> Terminator/1
  V_ROAD_REF/1 -> [ASMBUS_Env_Driver_vRef]
  Reduce_Dimension4/1(Out) -> V_ROAD_REF/15
  Reduce_Dimension3/1(Out) -> V_ROAD_REF/14
  a_z_Max_Deflect[m|s2]/1 -> V_ROAD_REF/17
  a_z_Max_Rebound[m|s2]/1 -> V_ROAD_REF/16
  Bus Selector4/3 -> Reduce_Dimension4/1(In)  "<Pos_z_Preview_Road[m]>"
  Bus Selector4/2 -> Reduce_Dimension3/1(In)  "<Pitch_Preview_Road[deg]>"
  Bus Selector4/1 -> V_ROAD_REF/13  "<s_Veh_Road[m]>"
  Bus Selector3/2 -> V_ROAD_REF/12  "<AccBr_Mode[1Stim|2Driver]>"
  Bus Selector3/1 -> V_ROAD_REF/11  "<Reset_VehicleStates[0|1]>"
  Bus Selector5/2 -> UnitConversion4/1  "<Speed_Limit_Preview_Road[km|h]>"
  Bus Selector5/1 -> UnitConversion/1  "<Speed_Limit_Veh[km|h]>"
  Bus Selector8/1 -> V_ROAD_REF/1  "<AdaptVelocityToRoad_Mode[1Off|2On]>"
  Bus Selector8/5 -> V_ROAD_REF/5  "<a_y_Max[m|s2]>"
  Bus Selector8/4 -> V_ROAD_REF/4  "<a_x_Brake_Threshold[m|s2]>"
  Bus Selector8/3 -> V_ROAD_REF/3  "<a_x_Max[m|s2]>"
  UnitConversion1/1 -> V_ROAD_REF/6
  Bus Selector2/1 -> UnitConversion1/1  "<v_x_Vehicle[km|h]>"
  Bus Selector8/2 -> V_ROAD_REF/2  "<v_Vehicle_Ref_Maneuver[m|s]>"
  UnitConversion4/1 -> Reduce_Dimension2/1(In)
  UnitConversion/1 -> V_ROAD_REF/9
  VehicleDynamics_Signals/1 -> Bus Selector2/1
  Extend_Dimension/1(Out) -> s_Preview_vRef[m]/1
  Reduce_Dimension2/1(Out) -> V_ROAD_REF/10
  Curves_are_not_considered/1 -> v_Vehicle_Ref_Preview[m|s]/1
  Bus Selector1/1 -> Curves_are_not_considered/1  "<v_Vehicle_Ref_Preview_Maneuver[m|s]>"

== system ASM_Traffic_V2X_Complete_Model_2/MDL/Environment/Driver/SignalSelection ==
  Maneuver_Signals : Inport
  Pos_AccPedal[%] : Inport  Port=2
  Pos_BrakePedal[%] : Inport  Port=3
  Pos_ClutchPedal[%] : Inport  Port=4
  Gear[] : Inport  Port=5
  SelectorLever_Driver[-3T|-2P|-1R|0N|1D] : Inport  Port=6
  t_Preview_vRef[s] : Inport  Port=7
  Angle_SteeringWheel[deg] : Inport  Port=8
  ASMSignalCollector : Subsystem
  Bus Creator : BusCreator  Inputs=2
  Bus Creator2 : BusCreator  Inputs=9
  Bus Selector3 : BusSelector  OutputSignals=TipShiftSignals.SW_TipTronic[-1Down|0Off|1Up],StartButtonSignals,ParkingBrakeSignals
  Driver_Signals : Outport
  wires:
  t_Preview_vRef[s]/1 -> Bus Creator2/5  "t_Preview_vRef[s]"
  Bus Creator2/1 -> Driver_Signals/1, ASMSignalCollector/1(Driver_Signals)  "Driver"
  Bus Selector3/3 -> Bus Creator2/9  "<ParkingBrakeSignals>"
  Bus Selector3/1 -> Bus Creator/2  "<SW_TipTronic[-1Down|0Off|1Up]>"
  SelectorLever_Driver[-3T|-2P|-1R|0N|1D]/1 -> Bus Creator/1  "SelectorLever[-3T|-2P|-1R|0N|1D]"
  Bus Creator/1 -> Bus Creator2/7  "AutomaticTrmCtrlSignals"
  Pos_BrakePedal[%]/1 -> Bus Creator2/2  "Pos_BrakePedal[%]"
  Pos_AccPedal[%]/1 -> Bus Creator2/1  "Pos_AccPedal[%]"
  Bus Selector3/2 -> Bus Creator2/8  "<StartButtonSignals>"
  Pos_ClutchPedal[%]/1 -> Bus Creator2/3  "Pos_ClutchPedal[%]"
  Angle_SteeringWheel[deg]/1 -> Bus Creator2/6  "Angle_SteeringWheel[deg]"
  Gear[]/1 -> Bus Creator2/4  "Gear[]"
  Maneuver_Signals/1 -> Bus Selector3/1

== system ASM_Traffic_V2X_Complete_Model_2/MDL/Environment/Driver/Source_of_eGoCAR_Control_Conditions ==
  note: SteeringAngle
  note: Break
  note: Throttle
  In1 : Inport
  Throttle_Input_SIM : Inport  Port=2
  Break_Input_SIM : Inport  Port=3
  Steering_Input_SIM : Inport  Port=4
  eGOCAR_Speed_kmh : Inport  Port=5
  Break_Switch_Value : Constant
  Bus Selector : BusSelector  OutputSignals=signal1,signal2,signal3
  Steer_Decision_Conditions : Subsystem
  Steer_Switch_Value : Constant
  Switch_Break : Switch  Criteria=u2 > Threshold
  Switch_Steer : Switch  Criteria=u2 > Threshold
  Switch_Throtle : Switch  Criteria=u2 > Threshold
  Terminator1 : Terminator
  Throtle_Switch_Value : Constant
  Throttle : Outport
  Break : Outport  Port=2
  Steering : Outport  Port=3
  wires:
  In1/1 -> Bus Selector/1
  Bus Selector/3 -> Switch_Steer/3  "<signal3>"
  Bus Selector/2 -> Switch_Break/3  "<signal2>"
  Bus Selector/1 -> Switch_Throtle/3  "<signal1>"
  Throttle_Input_SIM/1 -> Switch_Throtle/1
  Throtle_Switch_Value/1 -> Switch_Throtle/2
  Break_Switch_Value/1 -> Switch_Break/2
  Steer_Switch_Value/1 -> Switch_Steer/2
  Steering_Input_SIM/1 -> Switch_Steer/1
  Break_Input_SIM/1 -> Switch_Break/1
  Switch_Throtle/1 -> Throttle/1
  Switch_Break/1 -> Break/1
  Switch_Steer/1 -> Steering/1
  eGOCAR_Speed_kmh/1 -> Steer_Decision_Conditions/1(In1)
  Steer_Decision_Conditions/1(Out1) -> Terminator1/1

== system ASM_Traffic_V2X_Complete_Model_2/MDL/Environment/Driver/SteeringWheelAngle_Control ==
  SteerWheelAngle_from_Sim : Inport
  Speed : Inport  Port=2
  Clock1 : Clock
  Ground : Ground
  steeringWheeelSelectionFunction : MATLAB Function  TreatAsAtomicUnit=on
  SteerWheelAngle : Outport
  wires:
  steeringWheeelSelectionFunction/1(strAngle) -> SteerWheelAngle/1
  SteerWheelAngle_from_Sim/1 -> steeringWheeelSelectionFunction/3(swaSim)
  Clock1/1 -> steeringWheeelSelectionFunction/1(clock)
  Ground/1 -> steeringWheeelSelectionFunction/4(swaFile)
  Speed/1 -> steeringWheeelSelectionFunction/2(speed)

== system ASM_Traffic_V2X_Complete_Model_2/MDL/Environment/EnvironmentInterface_In/Drivetrain ==
  Drivetrain : Inport
  Bus Selector5 : BusSelector  OutputSignals=Crankshaft.n_Engine[rpm],Transmission.ActiveTransmission.omega_Out_Trm[rad|s]
  Mapping : Subsystem
  Drivetrain_Signals : Outport
  wires:
  Bus Selector5/2 -> Mapping/2(omega_Out_Trm[rad|s]_)  "<omega_Out_Trm[rad|s]>"
  Bus Selector5/1 -> Mapping/1(n_Engine[rpm]_)  "<n_Engine[rpm]>"
  Mapping/1(Out) -> Drivetrain_Signals/1
  Drivetrain/1 -> Bus Selector5/1

== system ASM_Traffic_V2X_Complete_Model_2/MDL/Environment/EnvironmentInterface_In/SoftECU_Engine ==
  SoftECU : Inport
  Bus Selector8 : BusSelector  OutputSignals=SoftECU_Engine.IdleSpeedControl.Const_n_Engine_Idle_Set[rpm],SoftECU_Engine.EngineOperation.State_Engine[0|1|2|3|4],SoftECU_ACC.Controller_ACC.FCW[0Off|1On],SoftECU_ACC.Controller_ACC.AEB[0Off|1On]
  Mapping : Subsystem
  SoftECU_Signals : Outport
  wires:
  Bus Selector8/2 -> Mapping/2(State_Engine[0|1|2|3|4])  "<State_Engine[0|1|2|3|4]>"
  Bus Selector8/4 -> Mapping/4(AEB[0Off|1On])  "<AEB[0Off|1On]>"
  Bus Selector8/3 -> Mapping/3(FCW[0Off|1On])  "<FCW[0Off|1On]>"
  Mapping/1(Out) -> SoftECU_Signals/1
  SoftECU/1 -> Bus Selector8/1
  Bus Selector8/1 -> Mapping/1(Const_n_Engine_Idle_Set[rpm])  "<Const_n_Engine_Idle_Set[rpm]>"

== system ASM_Traffic_V2X_Complete_Model_2/MDL/Environment/EnvironmentInterface_In/Steering ==
  Steering : Inport
  Bus Selector8 : BusSelector  OutputSignals=i_Steering_Mean[],Angle_SteeringWheel[deg],SteeringWheelTorque.Trq_SteeringWheel[Nm]
  Mapping : Subsystem
  Steering_Signals : Outport
  wires:
  Bus Selector8/3 -> Mapping/3(Trq_SteeringWheel[Nm])  "<Trq_SteeringWheel[Nm]>"
  Bus Selector8/2 -> Mapping/2(Angle_SteeringWheel[deg])  "<Angle_SteeringWheel[deg]>"
  Bus Selector8/1 -> Mapping/1(i_Steering_Mean[])  "<i_Steering_Mean[]>"
  Steering/1 -> Bus Selector8/1
  Mapping/1(Out) -> Steering_Signals/1

== system ASM_Traffic_V2X_Complete_Model_2/MDL/Environment/EnvironmentInterface_In/Tire ==
  Tire : Inport
  Bus Selector1 : BusSelector  OutputSignals=Tire_FL.ActiveTire.r_Dyn_FL_Tire[m],Tire_FR.ActiveTire.r_Dyn_FR_Tire[m],Tire_RL.ActiveTire.r_Dyn_RL_Tire[m],Tire_RR.ActiveTire.r_Dyn_RR_Tire[m],Tire_FL.ActiveTire.Coef_RollingRes_FL[],Tire_FR.ActiveTire.Coef_RollingRes_FR[],Tire_RL.ActiveTire.Coef_RollingRes_RL[],Tire_RR.ActiveTire.Coef_RollingRes_RR[],Tire_FL.ActiveTire.CorneringStiffness_FL[N],Tire_FR.ActiveTire.CorneringStiffness_FR[N],Tire_RL.ActiveTire.CorneringStiffness_RL[N],Tire_RR.ActiveTire.CorneringStiffness_RR[N],Tire_FL.ContactPoint.Pos_CP_FL_CoorSys_E[x;y][m],Tire_FR.ContactPoint.Pos_CP_FR_CoorSys_E[x;y][m],Tire_RL.ContactPoint.Pos_CP_RL_CoorSys_E[x;y][m],Tire_RR.ContactPoint.Pos_CP_RR_CoorSys_E[x;y][m]
  Coef_RolRes_Mean : Fcn  Expr=(u(1)+u(2)+u(3)+u(4))/4
  CornStiff_Front_Mean : Fcn  Expr=(u(1)+u(2))/2
  CornStiff_Rear_Mean : Fcn  Expr=(u(1)+u(2))/2
  Mapping : Subsystem
  Mux : Mux
  Mux1 : Mux
  Mux2 : Mux  Inputs=2
  Mux3 : Mux  Inputs=2
  r_Dyn_Tire_Mean : Fcn  Expr=(u(1)+u(2)+u(3)+u(4))/4
  Tire_Signals : Outport
  wires:
  Tire/1 -> Bus Selector1/1
  Mux1/1 -> Coef_RolRes_Mean/1
  Mux/1 -> r_Dyn_Tire_Mean/1
  r_Dyn_Tire_Mean/1 -> Mapping/1(r_Dyn_Tire_Mean[m])
  Coef_RolRes_Mean/1 -> Mapping/2(Coef_RollingRes_Mean[])
  Mux2/1 -> CornStiff_Front_Mean/1
  Mux3/1 -> CornStiff_Rear_Mean/1
  CornStiff_Front_Mean/1 -> Mapping/3(CorneringStiffness_Tire_Front[N|rad])
  CornStiff_Rear_Mean/1 -> Mapping/4(CorneringStiffness_Tire_Rear[N|rad])
  Mapping/1(Out) -> Tire_Signals/1
  Bus Selector1/1 -> Mux/1  "<r_Dyn_FL_Tire[m]>"
  Bus Selector1/2 -> Mux/2  "<r_Dyn_FR_Tire[m]>"
  Bus Selector1/3 -> Mux/3  "<r_Dyn_RL_Tire[m]>"
  Bus Selector1/4 -> Mux/4  "<r_Dyn_RR_Tire[m]>"
  Bus Selector1/5 -> Mux1/1  "<Coef_RollingRes_FL[]>"
  Bus Selector1/6 -> Mux1/2  "<Coef_RollingRes_FR[]>"
  Bus Selector1/7 -> Mux1/3  "<Coef_RollingRes_RL[]>"
  Bus Selector1/8 -> Mux1/4  "<Coef_RollingRes_RR[]>"
  Bus Selector1/9 -> Mux2/1  "<CorneringStiffness_FL[N]>"
  Bus Selector1/10 -> Mux2/2  "<CorneringStiffness_FR[N]>"
  Bus Selector1/11 -> Mux3/1  "<CorneringStiffness_RL[N]>"
  Bus Selector1/12 -> Mux3/2  "<CorneringStiffness_RR[N]>"
  Bus Selector1/13 -> Mapping/5(Pos_CP_FL_CoorSys_E[x;y][m])  "<Pos_CP_FL_CoorSys_E[x;y][m]>"
  Bus Selector1/14 -> Mapping/6(Pos_CP_FR_CoorSys_E[x;y][m])  "<Pos_CP_FR_CoorSys_E[x;y][m]>"
  Bus Selector1/15 -> Mapping/7(Pos_CP_RL_CoorSys_E[x;y][m])  "<Pos_CP_RL_CoorSys_E[x;y][m]>"
  Bus Selector1/16 -> Mapping/8(Pos_CP_RR_CoorSys_E[x;y][m])  "<Pos_CP_RR_CoorSys_E[x;y][m]>"

== system ASM_Traffic_V2X_Complete_Model_2/MDL/Environment/EnvironmentInterface_In/VehicleMovement ==
  VehicleMovement : Inport
  Aerodynamics : Inport  Port=2
  Bus Creator : BusCreator  Inputs=5
  Bus Selector1 : BusSelector  OutputSignals=Forces.F_x_Aero_CoorSys_V[N]
  Bus Selector2 : BusSelector  OutputSignals=Vehicle.Linear.Pos_Vehicle_CoorSys_E[x;y;z][m],Vehicle.Angular.Angle_Vehicle_CoorSys_E[x;y;z][deg],Vehicle.Linear.s_Vehicle[m],Vehicle.Angular.RotationMatrix_V_to_E[3x3]
  Bus Selector5 : BusSelector  OutputSignals=Positions,Velocities,Accelerations,VehicleMassAndAdditionalLoads,MassForcesAndTorques.GravitationalForces.F_Vehicle_Gravitational[x;y;z][N]
  Bus Selector7 : BusSelector  OutputSignals=VehicleCoG.Linear.a_Vehicle_CoG[x;y;z][m|s2].a_y_Vehicle_CoG[m|s2]
  Bus Selector8 : BusSelector  OutputSignals=Vehicle.Linear.v_Vehicle_CoG[x;y;z][km|h].v_x_Vehicle_CoG[km|h],Vehicle.Linear.v_Vehicle_CoG[x;y;z][km|h].v_y_Vehicle_CoG[km|h],Vehicle.Angular.w_Vehicle_CoG[x;y;z][deg|s].RollRate_Vehicle_CoG[deg|s],Vehicle.Angular.w_Vehicle_CoG[x;y;z][deg|s].YawRate_Vehicle_CoG[deg|s]
  Bus Selector9 : BusSelector  OutputSignals=m_TotalVehicle[kg],PosVec_CoG_TotalVehicle[x;y;z][m],Inertia_Tensor_TotalVehicle[3x3][kgm2]
  Mapping : Subsystem
  Mapping_Acc : Subsystem
  Mapping_F : Subsystem
  Mapping_Pos : Subsystem
  Mapping_Vel : Subsystem
  Selector_Inertia_z : Selector  NumberOfDimensions=2  InputPortWidth=3  IndexOptions=Index vector (dialog),Index vector (dialog)  Indices=3,3  OutputSizes=1
  Selector_Pos_x_COG : Selector  InputPortWidth=3  IndexOptions=Index vector (dialog)  Indices=[1]  OutputSizes=1
  X_Component : Selector  InputPortWidth=3  IndexOptions=Index vector (dialog)  Indices=[1]  OutputSizes=1
  Z_Component : Selector  InputPortWidth=3  IndexOptions=Index vector (dialog)  Indices=[3]  OutputSizes=1
  VehicleMovement_Signals : Outport
  wires:
  Bus Selector5/5 -> Z_Component/1, X_Component/1  "<F_Vehicle_Gravitational[x;y;z][N]>"
  Bus Selector1/1 -> Mapping_F/3(F_x_Aero_CoorSys_V[N])  "<F_x_Aero_CoorSys_V[N]>"
  Aerodynamics/1 -> Bus Selector1/1
  Z_Component/1 -> Mapping_F/2(F_z_Vehicle_Gravitational[N])
  X_Component/1 -> Mapping_F/1(F_x_Vehicle_Gravitational[N])
  Mapping_F/1(Out) -> Bus Creator/5
  Bus Selector2/4 -> Mapping_Pos/4(RotationMatrix_V_to_E[3x3])  "<RotationMatrix_V_to_E[3x3]>"
  Bus Selector5/1 -> Bus Selector2/1  "<Positions>"
  Bus Selector2/1 -> Mapping_Pos/1(Pos_Vehicle_CoorSys_E[x;y;z][m])  "<Pos_Vehicle_CoorSys_E[x;y;z][m]>"
  Bus Selector2/2 -> Mapping_Pos/2(Angle_Vehicle_CoorSys_E[x;y;z][deg])  "<Angle_Vehicle_CoorSys_E[x;y;z][deg]>"
  Bus Selector2/3 -> Mapping_Pos/3(s_Vehicle[m])  "<s_Vehicle[m]>"
  Selector_Inertia_z/1 -> Mapping/3(Inertia_z_Vehicle_Total[kgm2])
  Selector_Pos_x_COG/1 -> Mapping/2(Pos_x_CoG_Vehicle_Total[m])
  Bus Creator/1 -> VehicleMovement_Signals/1  "VehicleMovement"
  Bus Selector5/3 -> Bus Selector7/1  "<Accelerations>"
  Bus Selector5/2 -> Bus Selector8/1  "<Velocities>"
  Bus Selector5/4 -> Bus Selector9/1  "<VehicleMassAndAdditionalLoads>"
  VehicleMovement/1 -> Bus Selector5/1
  Mapping_Pos/1(Out) -> Bus Creator/1
  Mapping_Vel/1(Out) -> Bus Creator/2
  Mapping_Acc/1(Out) -> Bus Creator/3
  Mapping/1(Out) -> Bus Creator/4
  Bus Selector8/1 -> Mapping_Vel/1(v_x_Vehicle_CoG[km|h])  "<v_x_Vehicle_CoG[km|h]>"
  Bus Selector8/2 -> Mapping_Vel/2(v_y_Vehicle_CoG[km|h])  "<v_y_Vehicle_CoG[km|h]>"
  Bus Selector8/3 -> Mapping_Vel/3(RollRate_Vehicle_CoG[deg|s])  "<RollRate_Vehicle_CoG[deg|s]>"
  Bus Selector8/4 -> Mapping_Vel/4(YawRate_Vehicle_CoG[deg|s])  "<YawRate_Vehicle_CoG[deg|s]>"
  Bus Selector7/1 -> Mapping_Acc/1(a_y_Vehicle_CoG[m|s2])  "<a_y_Vehicle_CoG[m|s2]>"
  Bus Selector9/1 -> Mapping/1(m_TotalVehicle[kg])  "<m_TotalVehicle[kg]>"
  Bus Selector9/2 -> Selector_Pos_x_COG/1  "<PosVec_CoG_TotalVehicle[x;y;z][m]>"
  Bus Selector9/3 -> Selector_Inertia_z/1  "<Inertia_Tensor_TotalVehicle[3x3][kgm2]>"

== system ASM_Traffic_V2X_Complete_Model_2/MDL/Environment/Maneuver/ASMSignalCollector ==
  Bus Creator : BusCreator  Inputs=2
  tag scope: ASMBUS_Environment_Maneuver=global
  wires:
  [ASMBUS_Environment_ManeuverScheduler] -> Bus Creator/1
  Bus Creator/1 -> [ASMBUS_Environment_Maneuver]  "Maneuver"
  [ASMBUS_Environment_Mnvr_UserSignalsCustomized] -> Bus Creator/2

== system ASM_Traffic_V2X_Complete_Model_2/MDL/Environment/Maneuver/Customize_UserSignals ==
  UserSignals_In : Inport
  Bus Creator : BusCreator  Inputs=8
  Bus Selector1 : BusSelector  OutputSignals=User1[],User2[],User3[],User4[],User5[],User6[],User7[],User8[]
  CustomizedUserSignals : Subsystem
  ASMSignalBus : Outport
  UserSignals_Customized : Outport  Port=2
  wires:
  CustomizedUserSignals/8(Mnv_DataStream_8[]) -> Bus Creator/8
  CustomizedUserSignals/7(Mnv_DataStream_7[]) -> Bus Creator/7
  CustomizedUserSignals/6(Mnv_DataStream_6[]) -> Bus Creator/6
  CustomizedUserSignals/5(Mnv_DataStream_5[]) -> Bus Creator/5
  Bus Selector1/8 -> CustomizedUserSignals/8(User8[])  "<User8[]>"
  Bus Selector1/7 -> CustomizedUserSignals/7(User7[])  "<User7[]>"
  Bus Selector1/6 -> CustomizedUserSignals/6(User6[])  "<User6[]>"
  Bus Selector1/5 -> CustomizedUserSignals/5(User5[])  "<User5[]>"
  Bus Selector1/4 -> CustomizedUserSignals/4(User4[])  "<User4[]>"
  Bus Selector1/3 -> CustomizedUserSignals/3(User3[])  "<User3[]>"
  CustomizedUserSignals/3(ASM_Vehicle_TurnLights[]) -> Bus Creator/3
  CustomizedUserSignals/4(ECU_Commands[]) -> Bus Creator/4
  UserSignals_In/1 -> Bus Selector1/1
  Bus Creator/1 -> UserSignals_Customized/1, ASMSignalBus/1  "UserSignals_Customized"
  Bus Selector1/1 -> CustomizedUserSignals/1(User1[])  "<User1[]>"
  Bus Selector1/2 -> CustomizedUserSignals/2(User2[])  "<User2[]>"
  CustomizedUserSignals/1(ExternalSegmentEnd_Mode[]) -> Bus Creator/1
  CustomizedUserSignals/2(ExternalSegmentEnd_Value[]) -> Bus Creator/2

== system ASM_Traffic_V2X_Complete_Model_2/MDL/Environment/Maneuver/ExternalSegmentEnd ==
  Road_Signals : Inport
  VehicleDynamics_Signals : Inport  Port=2
  Traffic_Signals : Inport  Port=3
  SoftECU_Signals : Inport  Port=4
  UserSignals_Customized : Inport  Port=5
  AvoidAlgLoop{1..9} (9 alike) : Memory
  Bus Selector : BusSelector  OutputSignals=ExternalSegmentEnd_Mode[],ExternalSegmentEnd_Value[]
  Bus Selector1 : BusSelector  OutputSignals=FellowMovement.UserSignals_Customized.ManeuverSegmentEndTrigger[0|1]
  Bus Selector2 : BusSelector  OutputSignals=Road_ASMVeh.s_Veh_Road[m]
  Bus Selector3 : BusSelector  OutputSignals=SensorOutput.Dist_Object[m]
  Bus Selector4 : BusSelector  OutputSignals=VehicleMovement.Velocities.RollRate_Vehicle[deg|s]
  Bus Selector5 : BusSelector  OutputSignals=SensorOutput.Dist_Object[m]
  Bus Selector6 : BusSelector  OutputSignals=SoftECU_ACC.FCW[0Off|1On],SoftECU_ACC.AEB[0Off|1On]
  Const_External_SegmentEnd_10[0|1] : Constant  Value=0
  Const_External_SegmentEnd_11_25 : Constant  Value=zeros(15,1)
  Const_External_SegmentEnd_5[0|1] : Constant  Value=0
  Const_External_SegmentEnd_6[0|1] : Constant  Value=0
  Const_External_SegmentEnd_7[0|1] : Constant  Value=0
  Const_External_SegmentEnd_8[0|1] : Constant  Value=0
  Const_External_SegmentEnd_9[0|1] : Constant  Value=0
  Dist_Front_Min : Subsystem
  Dist_Rear_Min : Subsystem
  Mux : Mux  Inputs=[1 1 1 1 1 1 1 1 1 1 15]
  SegmentEndTrigger : Subsystem
  External_SegmentEnd[0|1] : Outport
  wires:
  AvoidAlgLoop9/1 -> Mux/4
  AvoidAlgLoop8/1 -> Mux/3
  Bus Selector6/2 -> AvoidAlgLoop9/1  "<AEB[0Off|1On]>"
  Bus Selector6/1 -> AvoidAlgLoop8/1  "<FCW[0Off|1On]>"
  SoftECU_Signals/1 -> Bus Selector6/1
  Const_External_SegmentEnd_5[0|1]/1 -> Mux/5
  Const_External_SegmentEnd_6[0|1]/1 -> Mux/6
  Const_External_SegmentEnd_7[0|1]/1 -> Mux/7
  Const_External_SegmentEnd_8[0|1]/1 -> Mux/8
  Const_External_SegmentEnd_9[0|1]/1 -> Mux/9
  Const_External_SegmentEnd_10[0|1]/1 -> Mux/10
  Mux/1 -> External_SegmentEnd[0|1]/1
  Traffic_Signals/1 -> Bus Selector1/1  "ManeuverEndTrigger[0|1]"
  Bus Selector1/1 -> AvoidAlgLoop6/1  "<ManeuverSegmentEndTrigger[0|1]>"
  AvoidAlgLoop6/1 -> Mux/2
  UserSignals_Customized/1 -> Bus Selector/1
  Bus Selector/1 -> AvoidAlgLoop1/1  "<ExternalSegmentEnd_Mode[]>"
  Bus Selector/2 -> AvoidAlgLoop2/1  "<ExternalSegmentEnd_Value[]>"
  VehicleDynamics_Signals/1 -> Bus Selector4/1
  Bus Selector4/1 -> AvoidAlgLoop4/1  "<RollRate_Vehicle[deg|s]>"
  Road_Signals/1 -> Bus Selector2/1
  Bus Selector2/1 -> AvoidAlgLoop3/1  "<s_Veh_Road[m]>"
  AvoidAlgLoop1/1 -> SegmentEndTrigger/1(ExternalSegmentEnd_Mode[])
  AvoidAlgLoop2/1 -> SegmentEndTrigger/2(ExternalSegmentEnd_Value[])
  AvoidAlgLoop3/1 -> SegmentEndTrigger/3(s_Road[m])
  AvoidAlgLoop4/1 -> SegmentEndTrigger/4(RollRate_Vehicle[deg|s])
  [ASMBUS_Environment_Traffic_3DObjSensor1_SensorSignals] -> Bus Selector3/1
  Bus Selector3/1 -> Dist_Front_Min/1(Dist_Front[m])  "<Dist_Object[m]>"
  [ASMBUS_Environment_Traffic_3DObjSensor3_SensorSignals] -> Bus Selector5/1
  Dist_Front_Min/1(Out1) -> AvoidAlgLoop5/1
  Bus Selector5/1 -> Dist_Rear_Min/1(Dist_Rear[m])  "<Dist_Object[m]>"
  Dist_Rear_Min/1(Out1) -> AvoidAlgLoop7/1
  AvoidAlgLoop7/1 -> SegmentEndTrigger/6(Distance_Rear[m])
  AvoidAlgLoop5/1 -> SegmentEndTrigger/5(Distance_Front[m])
  SegmentEndTrigger/1(External_SegmentEnd[0|1]) -> Mux/1
  Const_External_SegmentEnd_11_25/1 -> Mux/11

== system ASM_Traffic_V2X_Complete_Model_2/MDL/Environment/Maneuver/ExternalUserData ==
  Angle_SteeringWheel[deg] : Constant  Value=0
  Bus Creator2 : BusCreator  Inputs=10
  Gear[] : Constant  Value=0
  LaneIdx_Ref[] : Constant  Value=0
  Pos_AccPedal[%] : Constant  Value=0
  Pos_BrakePedal[%] : Constant  Value=0
  Pos_ClutchPedal[%] : Constant  Value=100
  "SelectorLever[] " : Constant  Value=0
  Trq_Steering[Nm] : Constant  Value=0
  d_Ref[m] : Constant  Value=0
  v_Vehicle_Ref[m|s] : Constant  Value=0
  External_ReferenceSignals : Outport
  wires:
  "SelectorLever[] "/1 -> Bus Creator2/10  "SelectorLever[]"
  Trq_Steering[Nm]/1 -> Bus Creator2/9  "Trq_Steering[Nm]"
  Angle_SteeringWheel[deg]/1 -> Bus Creator2/5  "Angle_SteeringWheel[deg]"
  Gear[]/1 -> Bus Creator2/4  "Gear[]"
  Pos_ClutchPedal[%]/1 -> Bus Creator2/3  "Pos_ClutchPedal[%]"
  Pos_BrakePedal[%]/1 -> Bus Creator2/2  "Pos_BrakePedal[%]"
  Pos_AccPedal[%]/1 -> Bus Creator2/1  "Pos_AccPedal[%]"
  v_Vehicle_Ref[m|s]/1 -> Bus Creator2/6  "v_Vehicle_Ref[m|s]"
  d_Ref[m]/1 -> Bus Creator2/7  "d_Ref[m]"
  LaneIdx_Ref[]/1 -> Bus Creator2/8  "LaneIdx_Ref[]"
  Bus Creator2/1 -> External_ReferenceSignals/1
